simulink model "massDamper"  (R2021a)
settings: Solver=VariableStepAuto  StartTime=0.0  StopTime=10.0  RelTol=1e-3
values from neighbouring files (symbols this model uses):
  b = 0.1    [ex02_dpa_mass.m]    (also in run_simulink_simulation.m; simulink_state_update_fn.m)
  m = 1    [ex02_dpa_mass.m]    (also in run_simulink_simulation.m; simulink_state_update_fn.m)
  x1_0 = 0    [ex02_dpa_mass.m]    (also in simulink_state_update_fn.m = X1(i, j))
  x2_0 = 0    [ex02_dpa_mass.m]    (also in simulink_state_update_fn.m = X2(i, j))
settings Model: Creator=adekoyoa  LastModifiedBy=adekoyoa

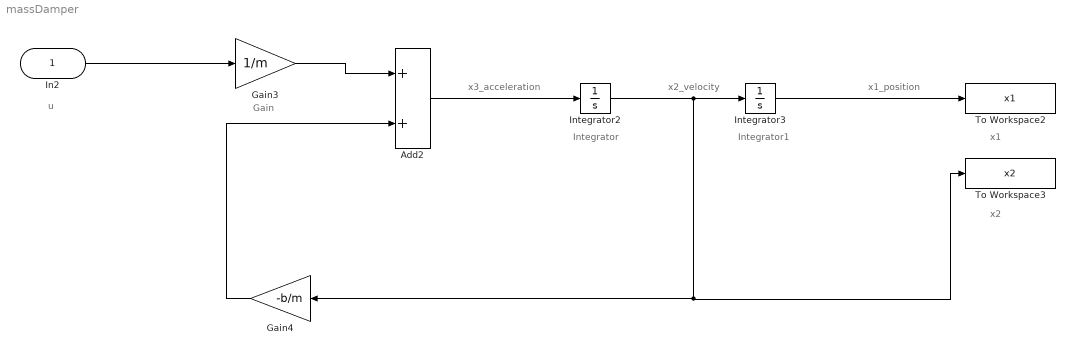
== system massDamper ==
  note: x3_acceleration
  note: x2_velocity
  note: Integrator
  note: x1_position
  note: Integrator1
  note: x2
  note: x1
  note: u
  note: Gain
  In2 : Inport
  Add2 : Sum
  Gain3 : Gain  Gain=1/m
  Gain4 : Gain  Gain=-b/m
  Integrator2 : Integrator  InitialCondition=x2_0
  Integrator3 : Integrator  InitialCondition=x1_0
  To Workspace2 : ToWorkspace  VariableName=x1  SampleTime=-1
  To Workspace3 : ToWorkspace  VariableName=x2  SampleTime=-1
  wires:
  Add2/1 -> Integrator2/1
  Integrator3/1 -> To Workspace2/1
  Integrator2/1 -> To Workspace3/1, Gain4/1, Integrator3/1
  Gain4/1 -> Add2/2
  Gain3/1 -> Add2/1
  In2/1 -> Gain3/1
